simulink model "Hopper_Model"  (R2020a)
settings: Solver=ode4  StartTime=0.0  StopTime=5  FixedStep=0.0005  RelTol=1e-3  EnableMultiTasking=on
settings Model: Creator=Cason  LastModifiedBy=Cason

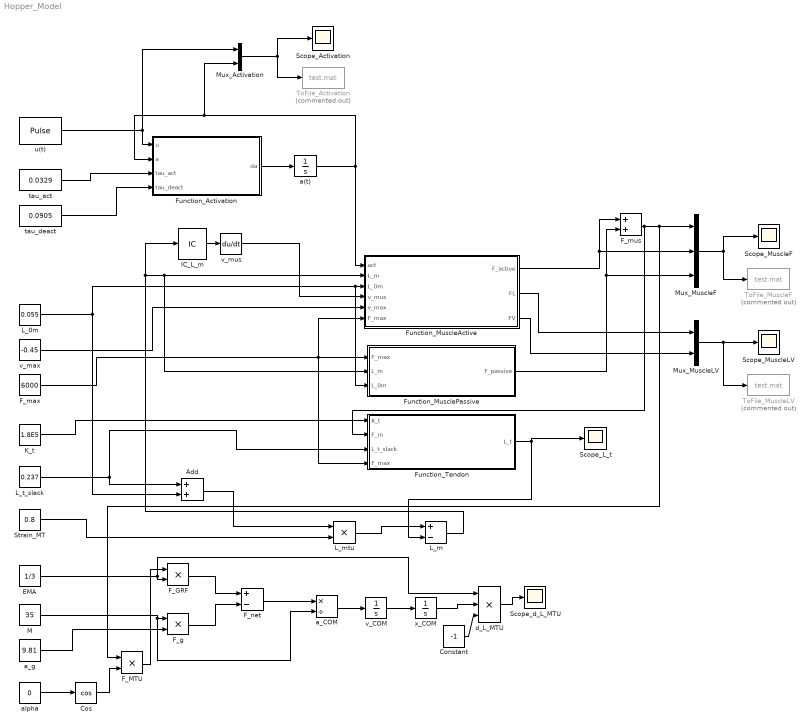
== system Hopper_Model ==
  Add : Sum
  Constant : Constant  Value=-1
  Cos : Trigonometry  Operator=cos
  EMA : Constant  Value=1/3
  F_GRF : Product
  F_MTU : Product
  F_g : Product
  F_max : Constant  Value=6000
  F_mus : Sum
  F_net : Sum  Inputs=+-
  Function_Activation : MATLAB Function  TreatAsAtomicUnit=on
  Function_MuscleActive : MATLAB Function  TreatAsAtomicUnit=on
  Function_MusclePassive : MATLAB Function  TreatAsAtomicUnit=on
  Function_Tendon : MATLAB Function  TreatAsAtomicUnit=on
  IC_L_m : InitialCondition  Value=0.055
  K_t : Constant  Value=1.8E5
  L_0m : Constant  Value=0.055
  L_m : Sum  Inputs=+-
  L_mtu : Product
  L_t_slack : Constant  Value=0.237
  M : Constant  Value=35
  Mux_Activation : Mux  Inputs=2
  Mux_MuscleF : Mux  Inputs=3
  Mux_MuscleLV : Mux  Inputs=2
  Scope_Activation : Scope
  Scope_L_t : Scope
  Scope_MuscleF : Scope
  Scope_MuscleLV : Scope
  Scope_d_L_MTU : Scope
  Strain_MT : Constant  Value=0.8
  ToFile_Activation : ToFile  Commented=on  Filename=test.mat  MatrixName=out
  ToFile_MuscleF : ToFile  Commented=on  Filename=test.mat  MatrixName=out
  ToFile_MuscleLV : ToFile  Commented=on  Filename=test.mat  MatrixName=out
  a(t) : Integrator
  a_COM : Product  Inputs=*/
  a_g : Constant  Value=9.81
  alpha : Constant  Value=0
  d_L_MTU : Product  Inputs=3
  tau_act : Constant  Value=0.0329
  tau_deact : Constant  Value=0.0905
  u(t) : DiscretePulseGenerator  PulseType=Time based  Period=1  PulseWidth=30  PhaseDelay=0.5
  v_COM : Integrator
  v_max : Constant  Value=-0.45
  v_mus : Derivative
  x_COM : Integrator
  wires:
  u(t)/1 -> Mux_Activation/1, Function_Activation/1(u)
  Function_Activation/1(da) -> a(t)/1
  a(t)/1 -> Mux_Activation/2, Function_Activation/2(a), Function_MuscleActive/1(act)
  tau_act/1 -> Function_Activation/3(tau_act)
  tau_deact/1 -> Function_Activation/4(tau_deact)
  Mux_Activation/1 -> Scope_Activation/1, ToFile_Activation/1
  v_max/1 -> Function_MuscleActive/5(v_max)
  F_max/1 -> Function_MusclePassive/1(F_max), Function_MuscleActive/6(F_max), Function_Tendon/4(F_max)
  L_m/1 -> IC_L_m/1, Function_MusclePassive/2(L_m), Function_MuscleActive/2(L_m)
  v_mus/1 -> Function_MuscleActive/4(v_mus)
  Function_MuscleActive/1(F_active) -> Mux_MuscleF/2, F_mus/1
  Function_MusclePassive/1(F_passive) -> Mux_MuscleF/3, F_mus/2
  Mux_MuscleF/1 -> ToFile_MuscleF/1, Scope_MuscleF/1
  Mux_MuscleLV/1 -> ToFile_MuscleLV/1, Scope_MuscleLV/1
  Function_MuscleActive/2(FL) -> Mux_MuscleLV/1
  Function_MuscleActive/3(FV) -> Mux_MuscleLV/2
  F_mus/1 -> Function_Tendon/2(F_m), F_MTU/1, Mux_MuscleF/1
  L_t_slack/1 -> Add/1, Function_Tendon/3(L_t_slack)
  K_t/1 -> Function_Tendon/1(K_t)
  Function_Tendon/1(L_t) -> L_m/2, Scope_L_t/1
  L_mtu/1 -> L_m/1
  Add/1 -> L_mtu/1
  IC_L_m/1 -> v_mus/1
  Strain_MT/1 -> L_mtu/2
  L_0m/1 -> Add/2, Function_MusclePassive/3(L_0m), Function_MuscleActive/3(L_0m)
  M/1 -> a_COM/2, F_g/1
  a_g/1 -> F_g/2
  EMA/1 -> F_GRF/2, d_L_MTU/1
  F_g/1 -> F_net/2
  F_GRF/1 -> F_net/1
  F_net/1 -> a_COM/1
  a_COM/1 -> v_COM/1
  v_COM/1 -> x_COM/1
  x_COM/1 -> d_L_MTU/2
  alpha/1 -> Cos/1
  Cos/1 -> F_MTU/2
  F_MTU/1 -> F_GRF/1
  d_L_MTU/1 -> Scope_d_L_MTU/1
  Constant/1 -> d_L_MTU/3

== matlab function Hopper_Model/Function_MuscleActive ==
  data: act input; F_active output; L_m input; L_0m input; v_mus input; v_max input; F_max input; FL output; FV output
function [F_active, FL, FV]= active_muscle_dynamics(act, L_m, L_0m, v_mus, v_max, F_max)
a = 3.1108; b = 0.8698; s = 0.3914;

if L_m < 0
    L_m = 0;
end

FL = exp(-abs(((L_m / L_0m)^b - 1) / s)^a);

if v_mus < v_max
    FV = 0;
elseif v_mus >= v_max && v_mus < 0  % Shortening
    FV = (1 - v_mus/v_max) / (1 + v_mus/(0.17*v_max));
else                                % Lengthening
    FV = 1.8 - 0.8*((1 + v_mus/v_max) / (1 - 7.56*(v_mus/(0.17*v_max))));
end

F_active = act * FL * FV * F_max;

== matlab function Hopper_Model/Function_Activation ==
  data: u input; da output; a input; tau_act input; tau_deact input
function da = activation(u, a, tau_act, tau_deact)
beta = tau_act / tau_deact;
da = u / tau_act - (beta + (1 - beta)*u) / tau_act * a;

== matlab function Hopper_Model/Function_MusclePassive ==
  data: F_max input; F_passive output; L_m input; L_0m input
function F_passive = passive_muscle_dynamics(F_max, L_m, L_0m)
A = 2.39E-2; b = 5.31;

F_passive = F_max*A*exp(b*(L_m/L_0m - 1));

== matlab function Hopper_Model/Function_Tendon ==
  data: K_t input; L_t output; F_m input; L_t_slack input; F_max input
function L_t = tendon_dynamics(K_t, F_m, L_t_slack, F_max)
D_L_t = (F_m + (F_max*log(-9*exp(-(20*F_m)/F_max)+ 10)) / 20) / K_t;
L_t = D_L_t + L_t_slack;
